simulink model "lab2q1blockdiagram"  (Simulink 8.7)
settings: Solver=ode45  StartTime=0.0  StopTime=3.0  RelTol=1e-3
settings Model: Creator=ALUNO  LastModifiedBy=gmcma
settings OptimizationCC: ExpressionDepthLimit=2147483647
settings DebuggingCC: SolverPrmCheckMsg=warning  StateNameClashWarn=warning

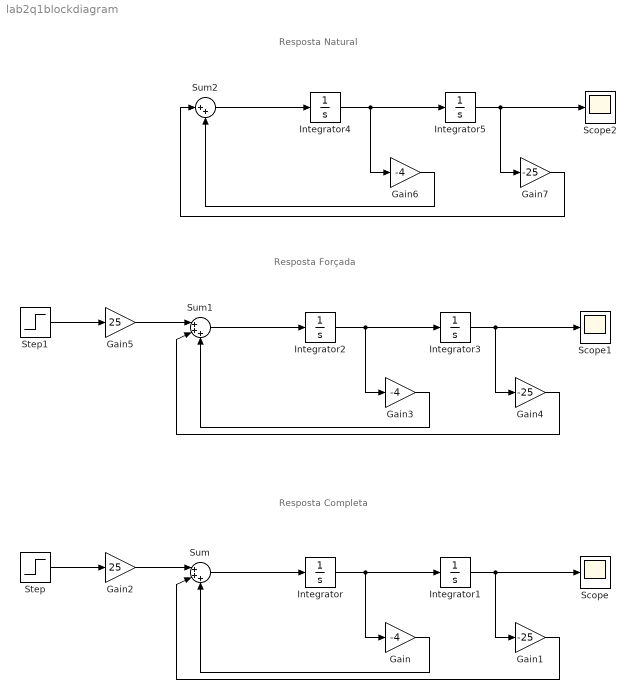
== system lab2q1blockdiagram ==
  note: Resposta Natural
  note: Resposta Forçada
  note: Resposta Completa
  Gain : Gain  Gain=-4
  Gain1 : Gain  Gain=-25
  Gain2 : Gain  Gain=25
  Gain3 : Gain  Gain=-4
  Gain4 : Gain  Gain=-25
  Gain5 : Gain  Gain=25
  Gain6 : Gain  Gain=-4
  Gain7 : Gain  Gain=-25
  Integrator : Integrator  InitialCondition=3
  Integrator1 : Integrator  InitialCondition=1
  Integrator2 : Integrator
  Integrator3 : Integrator
  Integrator4 : Integrator  InitialCondition=3
  Integrator5 : Integrator  InitialCondition=1
  Scope : Scope
  Scope1 : Scope
  Scope2 : Scope
  Step : Step  Time=0  SampleTime=0
  Step1 : Step  Time=0  SampleTime=0
  Sum : Sum  Inputs=|+++
  Sum1 : Sum  Inputs=|+++
  Sum2 : Sum  Inputs=|++
  wires:
  Step/1 -> Gain2/1
  Gain2/1 -> Sum/1
  Sum/1 -> Integrator/1
  Integrator/1 -> Gain/1, Integrator1/1
  Integrator1/1 -> Scope/1, Gain1/1
  Gain1/1 -> Sum/2
  Gain/1 -> Sum/3
  Step1/1 -> Gain5/1
  Gain5/1 -> Sum1/1
  Sum1/1 -> Integrator2/1
  Integrator2/1 -> Gain3/1, Integrator3/1
  Integrator3/1 -> Scope1/1, Gain4/1
  Gain4/1 -> Sum1/2
  Gain3/1 -> Sum1/3
  Sum2/1 -> Integrator4/1
  Integrator4/1 -> Gain6/1, Integrator5/1
  Integrator5/1 -> Scope2/1, Gain7/1
  Gain6/1 -> Sum2/2
  Gain7/1 -> Sum2/1
